simulink model "Problem1"  (R2020a)
settings: Solver=FixedStepAuto  StartTime=0.0  StopTime=10  FixedStep=0.001  RelTol=1e-3
model workspace (MAT data in the model file):
  B = 50
  K1 = 50
  K2 = 60
  M1 = 100
  M2 = 120
settings Model: Creator=tnradm  LastModifiedBy=tnradm

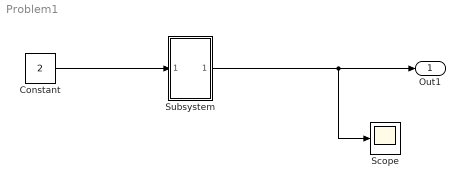
== system Problem1 ==
  Constant : Constant  Value=2
  Scope : Scope
  Subsystem : Subsystem  mask{M2=120, K2=50}
  Out1 : Outport
  wires:
  Constant/1 -> Subsystem/1(In1)
  Subsystem/1(Out1) -> Scope/1, Out1/1

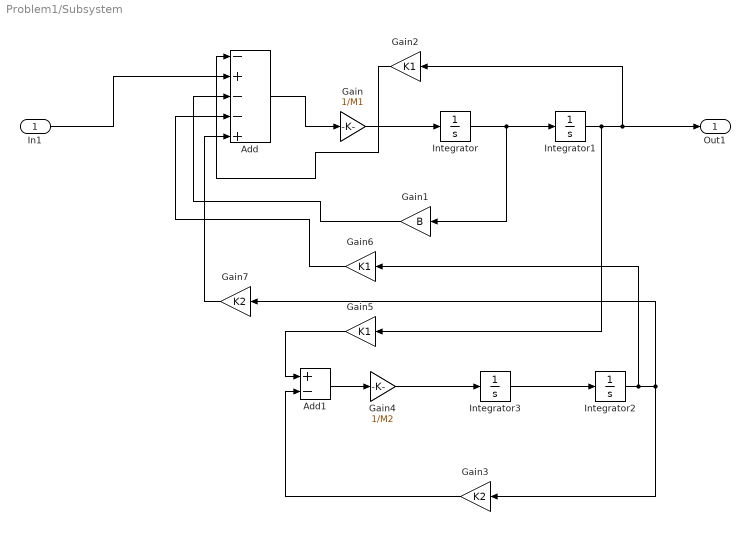
== system Problem1/Subsystem ==
  In1 : Inport
  Add : Sum  Inputs=-+--+
  Add1 : Sum  Inputs=+-
  Gain : Gain  Gain=1/M1
  Gain1 : Gain  Gain=B
  Gain2 : Gain  Gain=K1
  Gain3 : Gain  Gain=K2
  Gain4 : Gain  Gain=1/M2
  Gain5 : Gain  Gain=K1
  Gain6 : Gain  Gain=K1
  Gain7 : Gain  Gain=K2
  Integrator{,1..3} (4 alike) : Integrator
  Out1 : Outport
  wires:
  Integrator/1 -> Gain1/1, Integrator1/1
  Gain3/1 -> Add1/2
  Integrator3/1 -> Integrator2/1
  Gain1/1 -> Add/3
  Gain/1 -> Integrator/1
  In1/1 -> Add/2
  Gain2/1 -> Add/1
  Integrator1/1 -> Gain5/1, Out1/1, Gain2/1
  Gain4/1 -> Integrator3/1
  Add/1 -> Gain/1
  Add1/1 -> Gain4/1
  Integrator2/1 -> Gain6/1, Gain7/1, Gain3/1
  Gain5/1 -> Add1/1
  Gain6/1 -> Add/4
  Gain7/1 -> Add/5
